simulink model "OpenLoopBraking"  (R2022b)
settings: configuration reference "VehicleFixed10ms" (kept outside this file)
settings Model: DataDictionary=VirtualVehicleTemplate.sldd  ModifiedByFormat=The MathWorks, Inc.  Creator=The MathWorks, Inc.  LastModifiedBy=The MathWorks, Inc.
settings ConfigSetRef: SourceName=VehicleFixed10ms

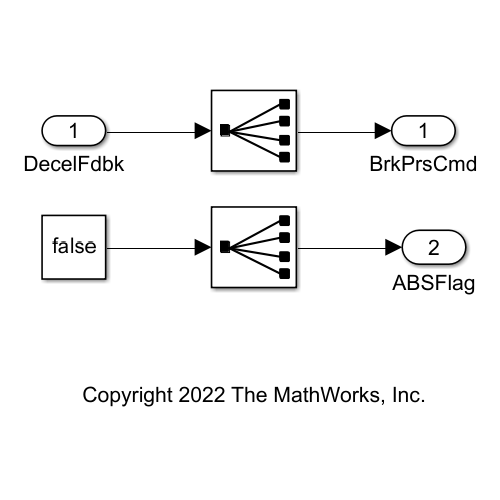
[thumbnail: Simulink's stored preview of the top-level diagram]
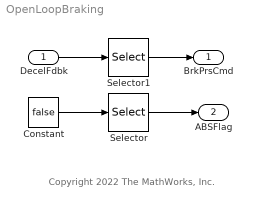
== system OpenLoopBraking ==
  note: Copyright 2022 The MathWorks, Inc.
  DecelFdbk : Inport  OutDataTypeStr=double  PortDimensions=1
  Constant : Constant  Value=false
  Selector : Selector  InputPortWidth=1  IndexOptions=Index vector (dialog)  Indices=[1 1 1 1]  OutputSizes=1
  Selector1 : Selector  InputPortWidth=1  IndexOptions=Index vector (dialog)  Indices=[1 1 1 1]  OutputSizes=1
  BrkPrsCmd : Outport  OutDataTypeStr=double  PortDimensions=4  VectorParamsAs1DForOutWhenUnconnected=off
  ABSFlag : Outport  Port=2  OutDataTypeStr=boolean  PortDimensions=4
  wires:
  Selector/1 -> ABSFlag/1
  Constant/1 -> Selector/1
  Selector1/1 -> BrkPrsCmd/1
  DecelFdbk/1 -> Selector1/1
